simulink model "p51_mass_spring_damper_sim"  (R2023a)
settings: Solver=VariableStepAuto  StartTime=0.0  StopTime=tf  MaxStep=1e-2  RelTol=1e-3
values from neighbouring files (symbols this model uses):
  b = 0.02    [p51_mass_spring_damper.m]
  k = 1    [p51_mass_spring_damper.m]
  M = 0.01    [p51_mass_spring_damper.m]
  x0 = [1; 0]    [p51_mass_spring_damper.m]
settings Model: Creator=alessandro  LastModifiedBy=admin
settings OptimizationCC: ReuseModelBlockBuffer=off

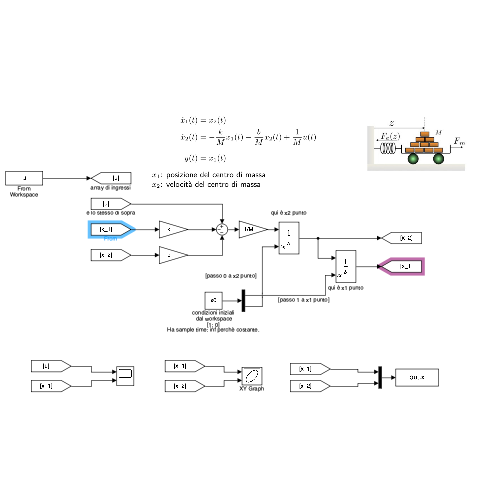
[thumbnail: Simulink's stored preview of the top-level diagram]
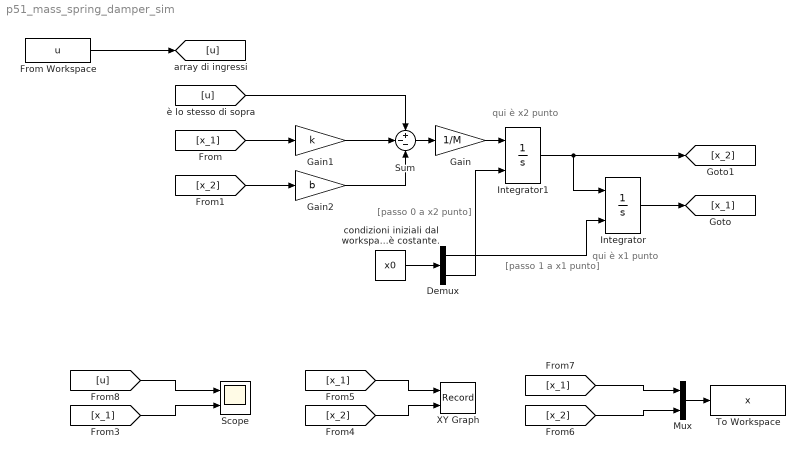
== system p51_mass_spring_damper_sim ==
  note: [passo 1 a x1 punto]
  note: qui è x1 punto
  note: qui è x2 punto
  note: [passo 0 a x2 punto]
  Demux : Demux  Outputs=2
  From Workspace : FromWorkspace  VariableName=u
  Gain : Gain  Gain=1/M
  Gain1 : Gain  Gain=k
  Gain2 : Gain  Gain=b
  Integrator : Integrator  InitialConditionSource=external
  Integrator1 : Integrator  InitialConditionSource=external
  Mux : Mux  Inputs=2
  Scope : Scope  NumInputPorts=2
  Sum : Sum  Inputs=+--
  To Workspace : ToWorkspace  VariableName=x  SaveFormat=Timeseries  SampleTime=-1
  XY Graph : Record  FileSettingsInternal="{\"entries\":[{\"content\":{\"excelSettings\":{\"content\":{},\"type\":\"Streamout.ExcelSettings\"}},\"type\":\"Streamout.FileSettingStorage\",\"uuid\":\"\"}],\"packageUris\":[\"http:\\/\\/schema.mathworks.com\\/mf0\\/streamout_blocks\\/R2020a\"],\"version\":\"1.0\"}"  Layout=[1 1]  SignalsInternal="{\"entries\":[{\"content\":{\"signals\":[{\"content\":{\"blockPath\":[],\"dimensions\":[1],\"domain\":\"\",\"lineColor\":\"#a2142f\",\"plots\":[1],\"port\":1,\"sid\":[\"\"],\"signalID\":144,\"signalName\":\"From5\"},\"type\":\"RecordBlkView.Signal\",\"uuid\":\"\"},{\"content\":{\"blockPath\":[],\"dimensions\":[1],\"domain\":\"\",\"lineColor\":\"#139fff\",\"plots\":[1],\"port\":2,\"sid\":[\"\"],\"signalID\":148,\"signalName\":\"From4\"},\"type\":\"RecordBlkView.Signal\",\"uuid\":\"\"}]},\"type\":\"RecordBlkView.InputSignals\",\"uuid\":\"\"}],\"packageUris\":[\"http:\\/\\/schema.mathworks.com\\/mf0\\/streamout_blocks\\/R2020a\"],\"version\":\"1.0\"}"  VisualizationBindings="{\"xyplotplugin\":{\"info\":[{\"series\":[{\"bindingParametersList\":[{\"parameter\":\"X-Axis\",\"signalID\":144,\"signalName\":\"From5\"},{\"parameter\":\"Y-Axis\",\"signalID\":148,\"signalName\":\"From4\"}],\"seriesID\":14036}],\"subplotID\":1}]}}"  CompatibilityTag=XY
  condizioni iniziali dal workspace [1; 0] Ha sample time: inf perchè costante. : Constant  Value=x0
  wires:
  Integrator/1 -> [x_1]
  Integrator1/1 -> Integrator/1, [x_2]
  condizioni iniziali dal workspace [1; 0] Ha sample time: inf perchè costante./1 -> Demux/1
  Demux/2 -> Integrator1/2
  Demux/1 -> Integrator/2
  Gain/1 -> Integrator1/1
  Sum/1 -> Gain/1
  [x_1] -> Gain1/1
  [x_2] -> Gain2/1
  Gain1/1 -> Sum/2
  Gain2/1 -> Sum/3
  [u] -> Sum/1
  From Workspace/1 -> [u]
  [x_1] -> Scope/2
  Mux/1 -> To Workspace/1
  [x_1] -> XY Graph/1
  [x_2] -> XY Graph/2
  [x_1] -> Mux/1
  [x_2] -> Mux/2
  [u] -> Scope/1
